simulink model "ohc_nonlinear_filter"  (R2020b)
settings: Solver=FixedStepDiscrete  StartTime=0.0  StopTime=stopTime  FixedStep=2.0833333333333333e-05  RelTol=1e-3
values from neighbouring files (symbols this model uses):
  minR = 0.5*R    [ohc_nonlinear_filter_parameters.m]
  taumax = 0.003    [modelparameters.m]
  taumin = 4.6310e-04    (= 0.0004631)    [modelparameters.m]
undefined symbols (not defined in the file or in its folder): s0
settings Model: Creator=Ross  LastModifiedBy=conno
settings DataIOCC: SaveOutput=off  SaveTime=off  ReturnWorkspaceOutputs=off
settings OptimizationCC: BlockReduction=off  ConditionallyExecuteInputs=off  DefaultParameterBehavior=Inlined
settings DebuggingCC: ReadBeforeWriteMsg=DisableAll  WriteAfterWriteMsg=DisableAll  WriteAfterReadMsg=DisableAll  AlgebraicLoopMsg=error  MultiTaskDSMMsg=none  SingleTaskRateTransMsg=error  PregeneratedLibrarySubsystemCodeDiagnostic=none  ArithmeticOperatorsInVariantConditions=warning
settings HardwareCC: ProdBitPerPointer=32  ProdBitPerSizeT=32  ProdBitPerPtrDiffT=32  ProdLargestAtomicFloat=None  ProdIntDivRoundTo=Undefined  ProdEndianess=Unspecified  ProdWordSize=32  ProdHWDeviceType=ASIC/FPGA->ASIC/FPGA  TargetBitPerPointer=64  TargetBitPerSizeT=64  TargetBitPerPtrDiffT=64  TargetLongLongMode=on  TargetIntDivRoundTo=Zero  TargetEndianess=LittleEndian  TargetWordSize=64  TargetHWDeviceType=Custom Processor->MATLAB Host Computer  ProdEqTarget=off
settings ModelReferenceCC: UpdateModelReferenceTargets=IfOutOfDate
settings SFSimCC: SFSimEcho=off  SimUseLocalCustomCode=off  CustomCodeUndefinedFunction=UseInterfaceOnly
settings RTWCC: RTWUseLocalCustomCode=off

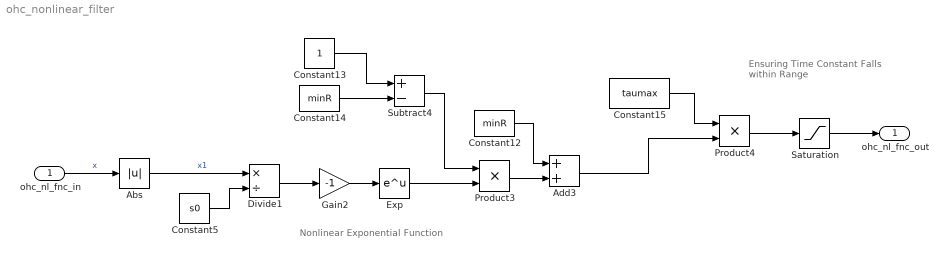
== system ohc_nonlinear_filter ==
  note: Ensuring Time Constant Falls within Range
  note: Nonlinear Exponential Function
  ohc_nl_fnc_in : Inport  OutDataTypeStr=single  PortDimensions=1  SampleTime=[2.0833333333333333e-05,0]
  Abs : Abs
  Add3 : Sum
  Constant12 : Constant  Value=minR  OutDataTypeStr=single  SampleTime=-1
  Constant13 : Constant  OutDataTypeStr=single  SampleTime=-1
  Constant14 : Constant  Value=minR  OutDataTypeStr=single  SampleTime=-1
  Constant15 : Constant  Value=taumax  OutDataTypeStr=single  SampleTime=-1
  Constant5 : Constant  Value=s0  OutDataTypeStr=single  SampleTime=-1
  Divide1 : Product  Inputs=*/  RndMeth=Zero  SaturateOnIntegerOverflow=on
  Exp : Math  SignedPower=on  SaturateOnIntegerOverflow=on
  Gain2 : Gain  Gain=-1
  Product3 : Product
  Product4 : Product
  Saturation : Saturate  UpperLimit=taumax  LowerLimit=taumin  OutDataTypeStr=single
  Subtract4 : Sum  Inputs=+-
  ohc_nl_fnc_out : Outport  OutDataTypeStr=single  PortDimensions=1  SampleTime=[2.0833333333333333e-05,0]  VectorParamsAs1DForOutWhenUnconnected=off
  wires:
  Saturation/1 -> ohc_nl_fnc_out/1
  Product4/1 -> Saturation/1
  Constant15/1 -> Product4/1
  Add3/1 -> Product4/2
  Constant12/1 -> Add3/1
  Constant14/1 -> Subtract4/2
  Product3/1 -> Add3/2
  Constant13/1 -> Subtract4/1
  Subtract4/1 -> Product3/1
  Abs/1 -> Divide1/1  "x1"
  Exp/1 -> Product3/2
  Divide1/1 -> Gain2/1
  ohc_nl_fnc_in/1 -> Abs/1  "x"
  Gain2/1 -> Exp/1
  Constant5/1 -> Divide1/2
